simulink model "EnvironmentMDL"  (R2020b)
settings: Solver=FixedStepAuto  StartTime=0.0  StopTime=10.0  RelTol=1e-3
undefined symbols (not defined in the file): initCond, km, s, vehicle, WMM2020
libraries: aerolibgravity2 x2, aerolibconvert2 x1, aerolibutil x1, aerolibcelestial x1
settings Model: Creator=dbell44  LastModifiedBy=dbell44

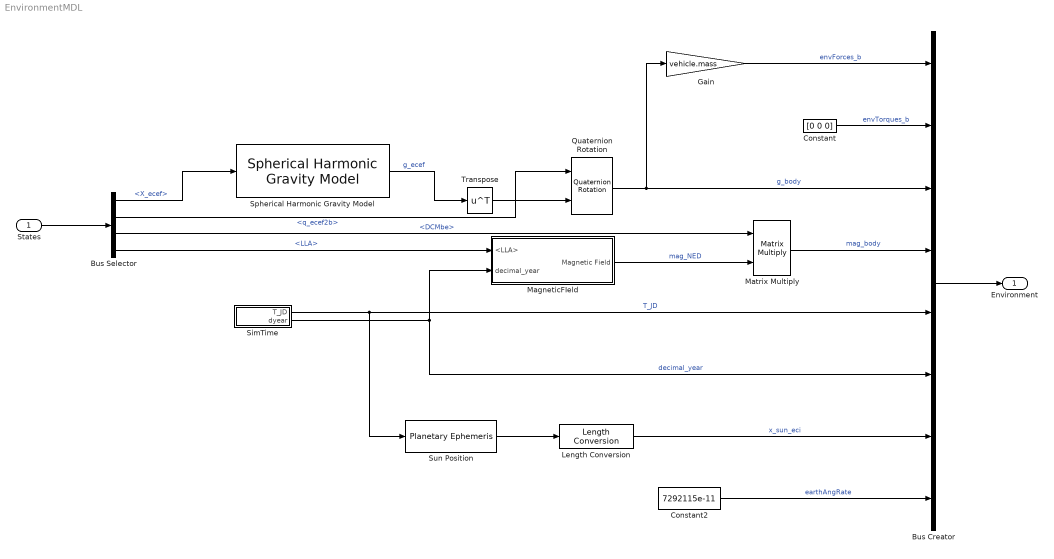
== system EnvironmentMDL ==
  States : Inport  OutDataTypeStr=Bus: States
  Bus Creator : BusCreator  Inputs=8
  Bus Selector : BusSelector  OutputSignals=X_ecef,q_ecef2b,DCMbe,LLA
  Constant : Constant  Value=[0 0 0]
  Constant2 : Constant  RequirementInfo={} %GIDa_a191e8b9_cb07_4d22_8813_52794fb76c2c  Value=7292115e-11
  Gain : Gain  Gain=vehicle.mass
  Length Conversion : aerolibconvert2/Length Conversion  IU=km  OU=m
  MagneticFIeld : Subsystem
  Matrix Multiply : Product  Multiplication=Matrix(*)
  Quaternion Rotation : aerolibutil/Quaternion Rotation
  SimTime : Subsystem
  Spherical Harmonic Gravity Model : aerolibgravity2/Spherical Harmonic Gravity Model  units=Metric (MKS)  degree=20  action=Warning  ptype=EGM2008  datafile='aerogmm2b.mat'
      settings: SourceProductBaseCode=AE
  Sun Position : aerolibcelestial/Planetary Ephemeris  kmflag=km,km/s  epochflag=Julian date  de=DE421  nCenter=Earth  nTarget=Sun  errorflag=Error  velflag=off
      settings: SourceProductBaseCode=AE
  Transpose : Math  Operator=transpose  SaturateOnIntegerOverflow=on
  Environment : Outport  OutDataTypeStr=Bus: Environment
  wires:
  Constant2/1 -> Bus Creator/8  "earthAngRate"
  Sun Position/1 -> Length Conversion/1
  Transpose/1 -> Quaternion Rotation/2
  Length Conversion/1 -> Bus Creator/7  "x_sun_eci"
  Bus Selector/2 -> Quaternion Rotation/1  "<q_ecef2b>"
  SimTime/2(dyear) -> MagneticFIeld/2(decimal_year), Bus Creator/6  "decimal_year"
  Bus Selector/4 -> MagneticFIeld/1(<LLA>)  "<LLA>"
  Bus Creator/1 -> Environment/1
  SimTime/1(T_JD) -> Bus Creator/5, Sun Position/1  "T_JD"
  Spherical Harmonic Gravity Model/1 -> Transpose/1  "g_ecef"
  Constant/1 -> Bus Creator/2  "envTorques_b"
  Matrix Multiply/1 -> Bus Creator/4  "mag_body"
  Quaternion Rotation/1 -> Gain/1, Bus Creator/3  "g_body"
  MagneticFIeld/1(Magnetic Field) -> Matrix Multiply/2  "mag_NED"
  Gain/1 -> Bus Creator/1  "envForces_b"
  States/1 -> Bus Selector/1
  Bus Selector/1 -> Spherical Harmonic Gravity Model/1  "<X_ecef>"
  Bus Selector/3 -> Matrix Multiply/1  "<DCMbe>"

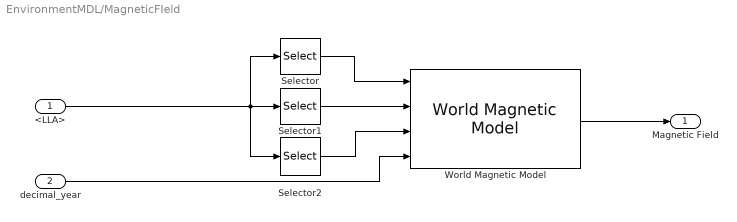
== system EnvironmentMDL/MagneticFIeld ==
  <LLA> : Inport
  decimal_year : Inport  Port=2
  Selector : Selector  InputPortWidth=3  IndexOptions=Index vector (dialog)  Indices=[3]  OutputSizes=1
  Selector1 : Selector  InputPortWidth=3  IndexOptions=Index vector (dialog)  Indices=[1]  OutputSizes=1
  Selector2 : Selector  InputPortWidth=3  IndexOptions=Index vector (dialog)  Indices=[2]  OutputSizes=1
  World Magnetic Model : aerolibgravity2/World Magnetic Model  model=WMM2020 (2020-2025)  customFile='WMM2020.COF'  units=Metric (MKS)  time_in=on  month=January  day=1  year=2020  action=Error  h_out=off  dec_out=off  inc_out=off  ti_out=off
      settings: SourceProductBaseCode=AE
  Magnetic Field : Outport
  wires:
  World Magnetic Model/1 -> Magnetic Field/1
  Selector/1 -> World Magnetic Model/1
  Selector1/1 -> World Magnetic Model/2
  Selector2/1 -> World Magnetic Model/3
  <LLA>/1 -> Selector2/1, Selector1/1, Selector/1
  decimal_year/1 -> World Magnetic Model/4

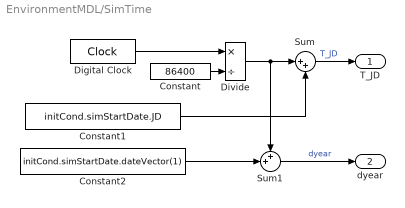
== system EnvironmentMDL/SimTime ==
  Constant : Constant  Value=86400
  Constant1 : Constant  Value=initCond.simStartDate.JD
  Constant2 : Constant  Value=initCond.simStartDate.dateVector(1)
  Digital Clock : DigitalClock
  Divide : Product  Inputs=*/
  Sum : Sum  Inputs=|++
  Sum1 : Sum  Inputs=++|
  T_JD : Outport
  dyear : Outport  Port=2
  wires:
  Sum/1 -> T_JD/1  "T_JD"
  Digital Clock/1 -> Divide/1
  Constant/1 -> Divide/2
  Divide/1 -> Sum/1, Sum1/1
  Sum1/1 -> dyear/1  "dyear"
  Constant2/1 -> Sum1/2
  Constant1/1 -> Sum/2
